simulink model "sf_bouncing"  (R2020a)
settings: Solver=VariableStepAuto  StartTime=0.0  StopTime=10.0  RelTol=1e-3
settings Model: Creator=bzhan  LastModifiedBy=bzhan

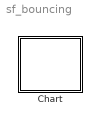
== system sf_bouncing ==
  Chart : Stateflow chart  TreatAsAtomicUnit=on

== stateflow chart sf_bouncing/Chart ==
  settings: updateMethod=CONTINUOUS
  state A
    du: x_dot=v; v_dot=a;
  (default) -> A : {x=5;v=0;a=-9.8;}
  A -> A : [x<=0&&v<=0]{v=-0.9*v;}
  data: v local; a local; x local
  data v settings: updateMethod=SF_CONTINUOUS_TIME_DATA
  data a settings: updateMethod=SF_CONTINUOUS_TIME_DATA
  data x settings: updateMethod=SF_CONTINUOUS_TIME_DATA
